simulink model "kinematic_model"  (Simulink 7.2)
settings: Solver=ode45  StartTime=0.0  StopTime=inf  RelTol=1e-3
values from neighbouring files (symbols this model uses):
  Brot = 0    [param_2224.m]
  Bwheel = 0    [param_2224.m]
  Dist_wheels = 0.12    [param_2224.m]
  Jrot = 2.7e-7    (= 2.7e-07)    [param_2224.m]
  Jwheel = 4.013e-6    (= 4.013e-06)    [param_2224.m]
  Ke = 1.115e-3*60/(2*pi)    (= 0.0106474656928)    [param_2224.m]
  Km = 11.12e-3    (= 0.01112)    [param_2224.m]
  L = 130e-6    (= 0.00013)    [param_2224.m]
  n = 8    [param_2224.m]
  R = 8.71    [param_2224.m]
  rads2mps = Rwheel*(2*pi)/(2*pi)    (= 0.0325)    [param_2224.m]
  rads2rpm = 60/(2*pi)    (= 9.54929658551)    [param_2224.m]
  ro = 0.9    [param_2224.m]
libraries: simulink x1
settings Model: Creator=void  LastModifiedBy=void
settings OptimizationCC: InlineInvariantSignals=on  InitFltsAndDblsToZero=on
settings DebuggingCC: SaveWithParameterizedLinksMsg=none  SignalResolutionControl=TryResolveAllWithWarning  MultiTaskDSMMsg=warning  MultiTaskCondExecSysMsg=none  StrictBusMsg=None
settings RTWCC: IncludeERTFirstTime=on
settings GRTTargetCC: TargetFcnLib=ansi_tfl_tmw.mat

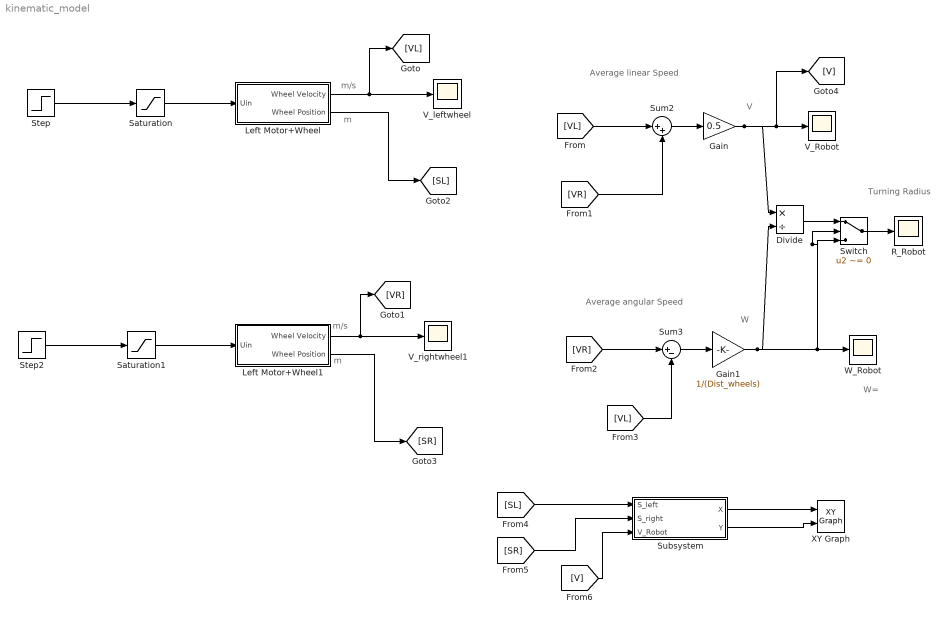
== system kinematic_model ==
  note: V
  note: W
  note: Average linear Speed
  note: Average angular Speed
  note: Turning Radius
  note: m/s
  note: m
  note: m/s
  note: m
  note: W=
  Divide : Product  Inputs=*/  OutDataType=sfix(16)  OutScaling=2^-10  SaturateOnIntegerOverflow=on
  Gain : Gain  Gain=0.5  ParameterDataType=sfix(16)  ParameterScaling=2^0  OutDataType=sfix(16)  OutScaling=2^0
  Gain1 : Gain  Gain=1/(Dist_wheels)  ParameterDataType=sfix(16)  ParameterScaling=2^0  OutDataType=sfix(16)  OutScaling=2^0
  Left Motor+Wheel : Subsystem
  Left Motor+Wheel1 : Subsystem
  R_Robot : Scope
      settings: TimeRange=1  YMin=0.969  YMax=1.071  SaveName=ScopeData5
  Saturation : Saturate  UpperLimit=11.1  LowerLimit=-11.1
  Saturation1 : Saturate  UpperLimit=11.1  LowerLimit=-11.1
  Step : Step  Time=0.3  After=8  SampleTime=0
  Step2 : Step  Time=0.3  After=9  SampleTime=0
  Subsystem : Subsystem
  Sum2 : Sum  Inputs=|++  OutDataType=sfix(16)  OutScaling=2^0
  Sum3 : Sum  Inputs=|+-  OutDataType=sfix(16)  OutScaling=2^0
  Switch : Switch  Criteria=u2 ~= 0
  V_Robot : Scope
      settings: TimeRange=1  YMin=3.2428  YMax=3.24317  SaveName=ScopeData3
  V_leftwheel : Scope
      settings: TimeRange=1.4  YMin=3.0495  YMax=3.0525
  V_rightwheel1 : Scope
      settings: TimeRange=1  YMin=3.43392  YMax=3.43393  SaveName=ScopeData2
  W_Robot : Scope
      settings: TimeRange=1  YMin=6.35911  YMax=6.35915  SaveName=ScopeData4
  XY Graph : simulink/Sinks/XY Graph  SystemSampleTime=-1  xmin=-3  xmax=3  ymin=-3  ymax=3  st=-1
  wires:
  Left Motor+Wheel/1(Wheel Velocity) -> [VL], V_leftwheel/1
  Saturation/1 -> Left Motor+Wheel/1(Uin)
  Step/1 -> Saturation/1
  Left Motor+Wheel1/1(Wheel Velocity) -> V_rightwheel1/1, [VR]
  Saturation1/1 -> Left Motor+Wheel1/1(Uin)
  Step2/1 -> Saturation1/1
  Sum2/1 -> Gain/1
  Gain/1 -> Divide/1, V_Robot/1, [V]
  [VL] -> Sum2/1
  [VR] -> Sum2/2
  Sum3/1 -> Gain1/1
  Gain1/1 -> Divide/2, W_Robot/1, Switch/3, Switch/2
  [VR] -> Sum3/1
  [VL] -> Sum3/2
  Divide/1 -> Switch/1
  Switch/1 -> R_Robot/1
  Left Motor+Wheel1/2(Wheel Position) -> [SR]
  Left Motor+Wheel/2(Wheel Position) -> [SL]
  Subsystem/1(X) -> XY Graph/1
  Subsystem/2(Y) -> XY Graph/2
  [SR] -> Subsystem/2(S_right)
  [V] -> Subsystem/3(V_Robot)
  [SL] -> Subsystem/1(S_left)

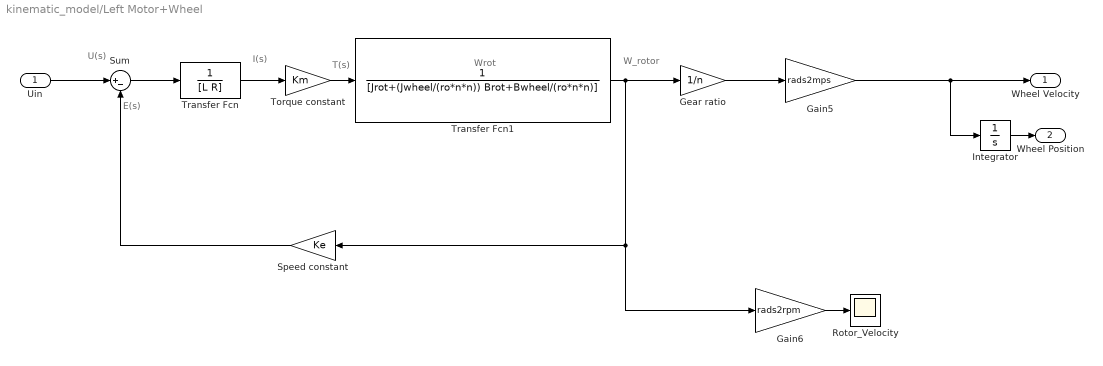
== system kinematic_model/Left Motor+Wheel ==
  note: I(s)
  note: E(s)
  note: U(s)
  note: T(s)
  note: Wrot
  note: W_rotor
  Uin : Inport  OutDataType=sfix(16)  OutScaling=2^0
  Gain5 : Gain  Gain=rads2mps  ParameterDataType=sfix(16)  ParameterScaling=2^0  OutDataType=sfix(16)  OutScaling=2^0
  Gain6 : Gain  Gain=rads2rpm  ParameterDataType=sfix(16)  ParameterScaling=2^0  OutDataType=sfix(16)  OutScaling=2^0
  Gear ratio : Gain  Gain=1/n  ParameterDataType=sfix(16)  ParameterScaling=2^0  OutDataType=sfix(16)  OutScaling=2^0
  Integrator : Integrator
  Rotor_Velocity : Scope
      settings: TimeRange=1  YMin=0.0025  YMax=0.0225
  Speed constant : Gain  Orientation=left  Gain=Ke  ParameterDataType=sfix(16)  ParameterScaling=2^0  OutDataType=sfix(16)  OutScaling=2^0
  Sum : Sum  Inputs=|+-  OutDataType=sfix(16)  OutScaling=2^0
  Torque constant : Gain  Gain=Km  ParameterDataType=sfix(16)  ParameterScaling=2^0  OutDataType=sfix(16)  OutScaling=2^0
  Transfer Fcn : TransferFcn  Denominator=[L R]
  Transfer Fcn1 : TransferFcn  Denominator=[Jrot+(Jwheel/(ro*n*n)) Brot+Bwheel/(ro*n*n)]
  Wheel Velocity : Outport  OutDataType=sfix(16)  OutScaling=2^0
  Wheel Position : Outport  Port=2  OutDataType=sfix(16)  OutScaling=2^0
  wires:
  Sum/1 -> Transfer Fcn/1
  Transfer Fcn/1 -> Torque constant/1
  Torque constant/1 -> Transfer Fcn1/1
  Speed constant/1 -> Sum/2
  Transfer Fcn1/1 -> Gear ratio/1, Speed constant/1, Gain6/1
  Gear ratio/1 -> Gain5/1
  Gain6/1 -> Rotor_Velocity/1
  Uin/1 -> Sum/1
  Gain5/1 -> Wheel Velocity/1, Integrator/1
  Integrator/1 -> Wheel Position/1

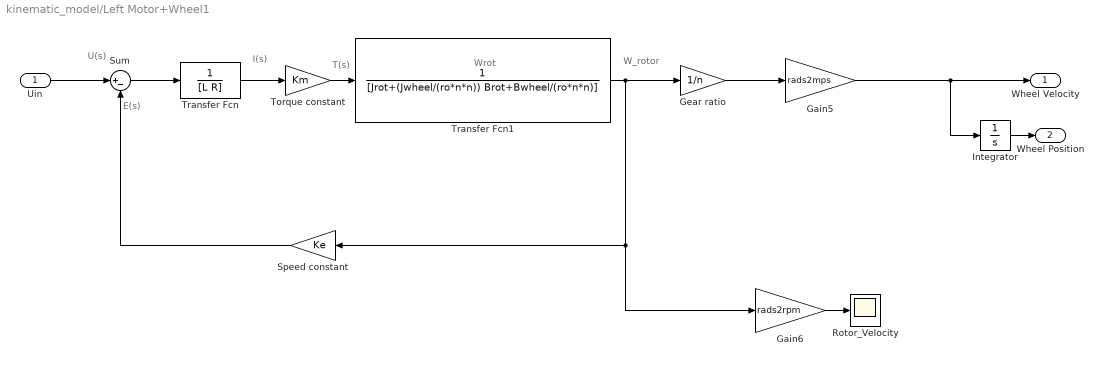
== system kinematic_model/Left Motor+Wheel1 ==
  note: I(s)
  note: E(s)
  note: U(s)
  note: T(s)
  note: Wrot
  note: W_rotor
  Uin : Inport  OutDataType=sfix(16)  OutScaling=2^0
  Gain5 : Gain  Gain=rads2mps  ParameterDataType=sfix(16)  ParameterScaling=2^0  OutDataType=sfix(16)  OutScaling=2^0
  Gain6 : Gain  Gain=rads2rpm  ParameterDataType=sfix(16)  ParameterScaling=2^0  OutDataType=sfix(16)  OutScaling=2^0
  Gear ratio : Gain  Gain=1/n  ParameterDataType=sfix(16)  ParameterScaling=2^0  OutDataType=sfix(16)  OutScaling=2^0
  Integrator : Integrator
  Rotor_Velocity : Scope
      settings: TimeRange=1  YMin=0.0025  YMax=0.0225
  Speed constant : Gain  Orientation=left  Gain=Ke  ParameterDataType=sfix(16)  ParameterScaling=2^0  OutDataType=sfix(16)  OutScaling=2^0
  Sum : Sum  Inputs=|+-  OutDataType=sfix(16)  OutScaling=2^0
  Torque constant : Gain  Gain=Km  ParameterDataType=sfix(16)  ParameterScaling=2^0  OutDataType=sfix(16)  OutScaling=2^0
  Transfer Fcn : TransferFcn  Denominator=[L R]
  Transfer Fcn1 : TransferFcn  Denominator=[Jrot+(Jwheel/(ro*n*n)) Brot+Bwheel/(ro*n*n)]
  Wheel Velocity : Outport  OutDataType=sfix(16)  OutScaling=2^0
  Wheel Position : Outport  Port=2  OutDataType=sfix(16)  OutScaling=2^0
  wires:
  Sum/1 -> Transfer Fcn/1
  Transfer Fcn/1 -> Torque constant/1
  Torque constant/1 -> Transfer Fcn1/1
  Speed constant/1 -> Sum/2
  Transfer Fcn1/1 -> Gear ratio/1, Speed constant/1, Gain6/1
  Gear ratio/1 -> Gain5/1
  Gain6/1 -> Rotor_Velocity/1
  Uin/1 -> Sum/1
  Gain5/1 -> Wheel Velocity/1, Integrator/1
  Integrator/1 -> Wheel Position/1

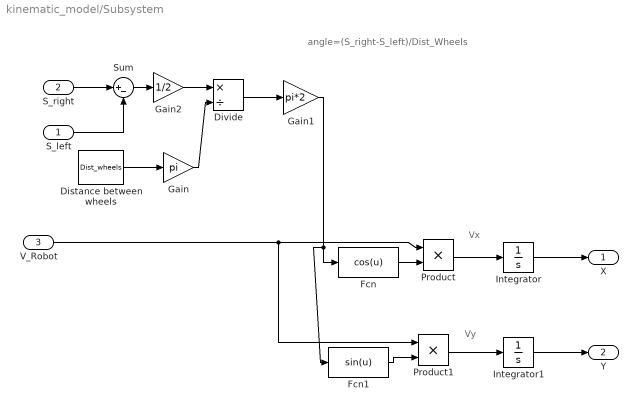
== system kinematic_model/Subsystem ==
  note: Vx
  note: Vy
  note: angle=(S_right-S_left)/Dist_Wheels
  S_left : Inport  OutDataType=sfix(16)  OutScaling=2^0
  S_right : Inport  Port=2  OutDataType=sfix(16)  OutScaling=2^0
  V_Robot : Inport  Port=3  OutDataType=sfix(16)  OutScaling=2^0
  Distance between wheels : Constant  Value=Dist_wheels  OutDataType=sfix(16)  OutScaling=2^0
  Divide : Product  Inputs=*/  OutDataType=sfix(16)  OutScaling=2^-10
  Fcn : Fcn  Expr=cos(u)
  Fcn1 : Fcn  Expr=sin(u)
  Gain : Gain  Gain=pi  ParameterDataType=sfix(16)  ParameterScaling=2^0  OutDataType=sfix(16)  OutScaling=2^0
  Gain1 : Gain  Gain=pi*2  ParameterDataType=sfix(16)  ParameterScaling=2^0  OutDataType=sfix(16)  OutScaling=2^0
  Gain2 : Gain  Gain=1/2  ParameterDataType=sfix(16)  ParameterScaling=2^0  OutDataType=sfix(16)  OutScaling=2^0
  Integrator : Integrator
  Integrator1 : Integrator
  Product : Product  OutDataType=sfix(16)  OutScaling=2^0  RndMeth=Zero
  Product1 : Product  OutDataType=sfix(16)  OutScaling=2^0  RndMeth=Zero
  Sum : Sum  Inputs=|+-  OutDataType=sfix(16)  OutScaling=2^0
  X : Outport  OutDataType=sfix(16)  OutScaling=2^0
  Y : Outport  Port=2  OutDataType=sfix(16)  OutScaling=2^0
  wires:
  Distance between wheels/1 -> Gain/1
  Gain/1 -> Divide/2
  Sum/1 -> Gain2/1
  Divide/1 -> Gain1/1
  Gain1/1 -> Fcn/1, Fcn1/1
  Fcn/1 -> Product/2
  Fcn1/1 -> Product1/2
  Product1/1 -> Integrator1/1
  V_Robot/1 -> Product1/1, Product/1
  Product/1 -> Integrator/1
  S_right/1 -> Sum/1
  S_left/1 -> Sum/2
  Gain2/1 -> Divide/1
  Integrator1/1 -> Y/1
  Integrator/1 -> X/1
